simulink model "PI_observador_ideal"  (R2021b)
settings: Solver=VariableStepAuto  StartTime=0.0  StopTime=40  RelTol=1e-3
undefined symbols (not defined in the file): A, B, C, K, ki
libraries: cstblocks x4
settings Model: Creator=axelt  LastModifiedBy=parra
settings DebuggingCC: UnconnectedInputMsg=none  UnconnectedOutputMsg=none  UnconnectedLineMsg=none
settings ModelReferenceCC: EnableRefExpFcnMdlSchedulingChecks=off
settings RTWCC: DLArmComputeVersion=20.02.1

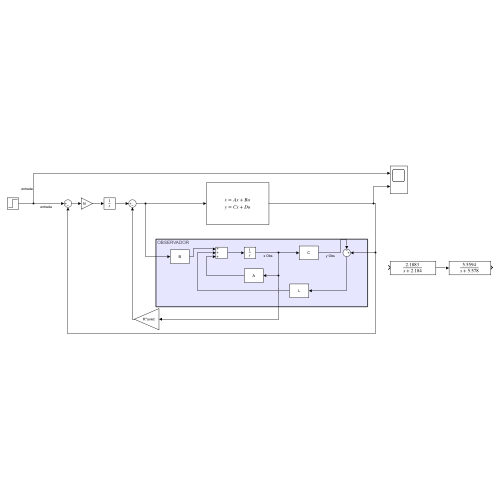
[thumbnail: Simulink's stored preview of the top-level diagram]
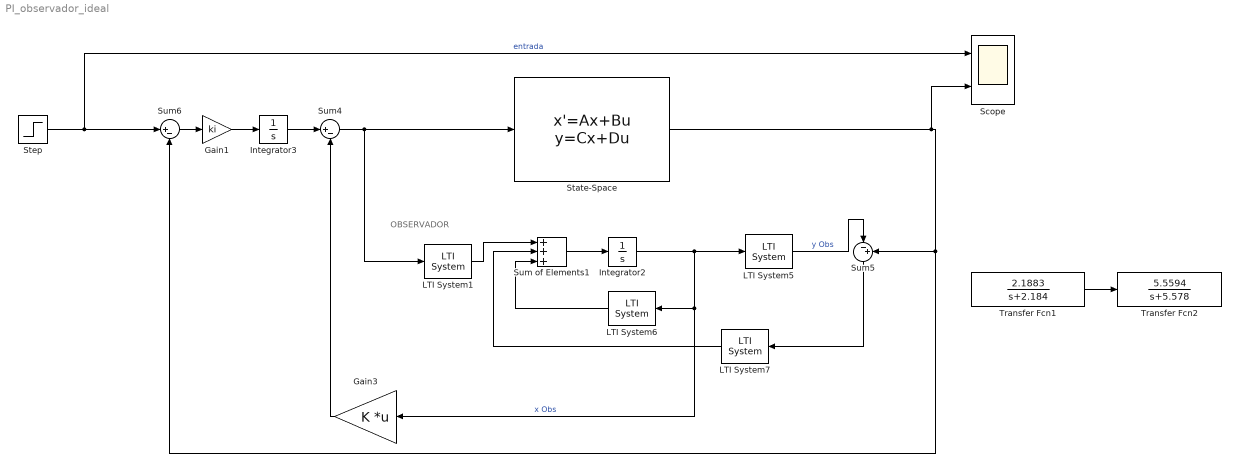
== system PI_observador_ideal ==
  note: OBSERVADOR
  Gain1 : Gain  Gain=ki
  Gain3 : Gain  Gain=K  Multiplication=Matrix(K*u) (u vector)
  Integrator2 : Integrator
  Integrator3 : Integrator
  LTI System1 : cstblocks/LTI System  sys=B  IC=[]
  LTI System5 : cstblocks/LTI System  sys=C  IC=[]
  LTI System6 : cstblocks/LTI System  sys=A  IC=[]
  LTI System7 : cstblocks/LTI System  sys=L  IC=[]
  Scope : Scope  NumInputPorts=2
  State-Space : StateSpace  A=A  B=B  C=C  D=0  InitialCondition=0
  Step : Step  Time=20  Before=0.5  SampleTime=0.01
  Sum of Elements1 : Sum  Inputs=+++
  Sum4 : Sum  Inputs=|+-
  Sum5 : Sum  Inputs=|-+
  Sum6 : Sum  Inputs=|+-
  Transfer Fcn1 : TransferFcn  Numerator=[2.1883]  Denominator=[1 2.184]
  Transfer Fcn2 : TransferFcn  Numerator=[5.5594]  Denominator=[1 5.578]
  wires:
  Gain1/1 -> Integrator3/1
  Integrator3/1 -> Sum4/1
  Sum5/1 -> LTI System7/1
  Gain3/1 -> Sum4/2
  Integrator2/1 -> LTI System5/1, LTI System6/1, Gain3/1  "x Obs"
  Step/1 -> Scope/1, Sum6/1  "entrada"
  Sum4/1 -> LTI System1/1, State-Space/1
  LTI System1/1 -> Sum of Elements1/1
  LTI System6/1 -> Sum of Elements1/3
  Sum of Elements1/1 -> Integrator2/1
  LTI System5/1 -> Sum5/1  "y Obs"
  Sum6/1 -> Gain1/1
  LTI System7/1 -> Sum of Elements1/2
  Transfer Fcn1/1 -> Transfer Fcn2/1
  State-Space/1 -> Scope/2, Sum5/2, Sum6/2
